simulink model "Practica2OscarModel"  (R2018a)
settings: Solver=VariableStepAuto  StartTime=0.0  StopTime=10.0  RelTol=1e-3  EnableMultiTasking=on
values from neighbouring files (symbols this model uses):
  K = 1.1    [Practica2Oscar.m]    (also in proyectoAvilaSilva.m = Kp/limite; proyectoAvilaSilva2.m = Kp/limite)
  Kd = Kv/lim    [P5OscarAvilaControlDigital.m]    (also in Practica2Oscar.m = 0.22; practica5.m = Kv/double(limit(f,s,0)))
  Kdv = 0.2    [Practica2Oscar.m]
  Ki = K*T/Ti    (= 0.2)    [Practica2Oscar.m]
  Kiv = 1.1    [Practica2Oscar.m]
  Kp = K-Ki/2    (= 1)    [Practica2Oscar.m]    (also in proyectoAvilaSilva.m = 9; proyectoAvilaSilva2.m = 9)
  Kpv = 5.5    [Practica2Oscar.m]
  T = 2.5    [P4OscarAvilaControlDigital.m]    (also in Practica2Oscar.m = 1; practica5.m = 0.02; proyectoAvilaSilva.m = 0.01; proyectoAvilaSilva2.m = 0.01)
  Td = 0.2    [Practica2Oscar.m]
  Ti = 5.5    [Practica2Oscar.m]
libraries: simulink x1
settings Model: Creator=CltControl  LastModifiedBy=sasm
settings OptimizationCC: LifeSpan=inf
settings DebuggingCC: SFUnexpectedBacktrackingDiag=warning  SFNoUnconditionalDefaultTransitionDiag=warning  SFExecutionAtInitializationDiag=none
settings CodeAppCC: StateflowObjectComments=on
settings GRTTargetCC: TargetLangStandard=C89/C90 (ANSI)  GeneratePreprocessorConditionals=Disable all
settings ConfigComp: CovMetricSettings=dw  CovHtmlReporting=on  CovSaveCumulativeToWorkspaceVar=on  CovSaveSingleToWorkspaceVar=on  CovExternalEMLEnable=off

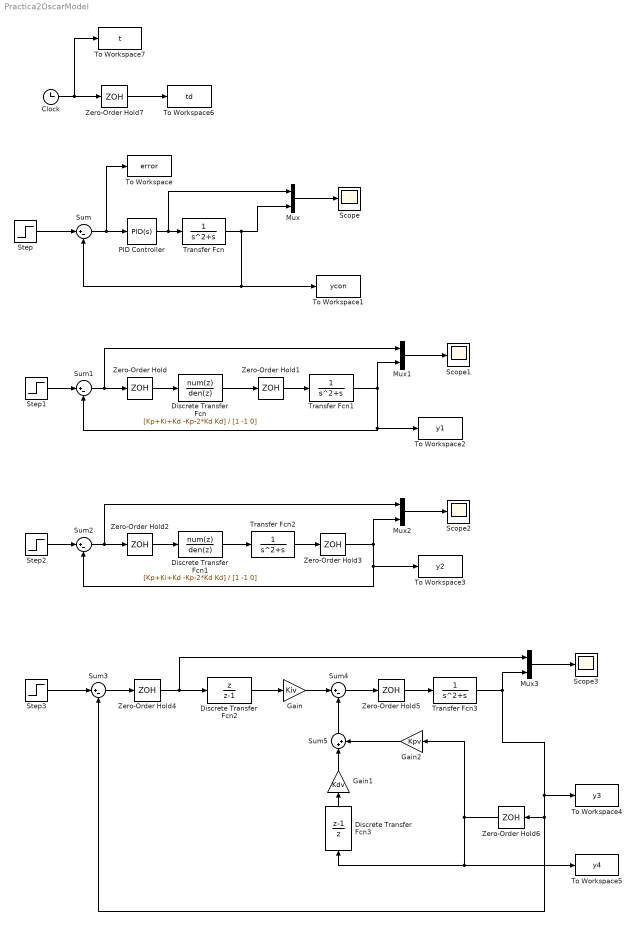
== system Practica2OscarModel ==
  Clock : Clock
  Discrete Transfer Fcn : DiscreteTransferFcn  Numerator=[Kp+Ki+Kd -Kp-2*Kd Kd]  Denominator=[1 -1 0]
  Discrete Transfer Fcn1 : DiscreteTransferFcn  Numerator=[Kp+Ki+Kd -Kp-2*Kd Kd]  Denominator=[1 -1 0]
  Discrete Transfer Fcn2 : DiscreteTransferFcn  Numerator=[1 0]  Denominator=[1 -1]
  Discrete Transfer Fcn3 : DiscreteTransferFcn  Numerator=[1 -1]  Denominator=[1 0]
  Gain : Gain  Gain=Kiv
  Gain1 : Gain  Gain=Kdv
  Gain2 : Gain  Gain=Kpv
  Mux{,1..3} (4 alike) : Mux  Inputs=2
  PID Controller : simulink/Continuous/PID Controller  Controller=PID  TimeDomain=Continuous-time  SampleTime=-1  IntegratorMethod=Forward Euler  FilterMethod=Forward Euler  Form=Ideal  UseFilter=on  ControllerParametersSource=internal  P=K  I=1/Ti  D=Td  N=100  InitialConditionSource=internal  InitialConditionForIntegrator=0  InitialConditionForFilter=0  ExternalReset=none  LimitOutput=off  UpperSaturationLimit=inf  LowerSaturationLimit=-inf  LinearizeAsGain=on  AntiWindupMode=none  Kb=1  TrackingMode=off  Kt=1  PParamMin=[]  PParamMax=[]  IParamMin=[]  IParamMax=[]  DParamMin=[]  DParamMax=[]  NParamMin=[]  NParamMax=[]  KbParamMin=[]  KbParamMax=[]  KtParamMin=[]  KtParamMax=[]  POutMin=[]  POutMax=[]  IOutMin=[]  IOutMax=[]  DOutMin=[]  DOutMax=[]  NOutMin=[]  NOutMax=[]  KbOutMin=[]  KbOutMax=[]  KtOutMin=[]  KtOutMax=[]  IntegratorOutMin=[]  IntegratorOutMax=[]  FilterOutMin=[]  FilterOutMax=[]  SumOutMin=[]  SumOutMax=[]  SumI1OutMin=[]  SumI1OutMax=[]  SumI2OutMin=[]  SumI2OutMax=[]  SumI3OutMin=[]  SumI3OutMax=[]  SumDOutMin=[]  SumDOutMax=[]  SaturationOutMin=[]  SaturationOutMax=[]  IntegratorContinuousStateAttributes=''  IntegratorStateMustResolveToSignalObject=off  IntegratorRTWStateStorageClass=Auto  FilterContinuousStateAttributes=''  FilterStateMustResolveToSignalObject=off  FilterRTWStateStorageClass=Auto  DifferentiatorICPrevScaledInput=0  DifferentiatorOutMin=[]  DifferentiatorOutMax=[]  FilterDiffOutCoefMin=[]  FilterDiffOutCoefMax=[]  SumDenOutMin=[]  SumDenOutMax=[]  SumNumOutMin=[]  SumNumOutMax=[]  ReciprocalOutMin=[]  ReciprocalOutMax=[]  DivideOutMin=[]  DivideOutMax=[]  TunerSelectOption=Transfer Function Based (PID Tuner App)
  Scope{,1..3} (4 alike) : Scope
  Step{,1..3} (4 alike) : Step  SampleTime=0
  Sum{,1..4} (5 alike) : Sum  Inputs=|+-
  Sum5 : Sum  Inputs=|++
  To Workspace : ToWorkspace  VariableName=error  SampleTime=-1
  To Workspace1 : ToWorkspace  VariableName=ycon  SampleTime=-1
  To Workspace2 : ToWorkspace  VariableName=y1  SampleTime=-1
  To Workspace3 : ToWorkspace  VariableName=y2  SampleTime=-1
  To Workspace4 : ToWorkspace  VariableName=y3  SampleTime=-1
  To Workspace5 : ToWorkspace  VariableName=y4  SampleTime=-1
  To Workspace6 : ToWorkspace  VariableName=td  SampleTime=-1
  To Workspace7 : ToWorkspace  VariableName=t  SampleTime=-1
  Transfer Fcn{,1..3} (4 alike) : TransferFcn  Denominator=[1 1 0]
  Zero-Order Hold{,1..7} (8 alike) : ZeroOrderHold  SampleTime=T
  wires:
  Step/1 -> Sum/1
  Sum/1 -> To Workspace/1, PID Controller/1
  PID Controller/1 -> Mux/1, Transfer Fcn/1
  Transfer Fcn/1 -> Sum/2, To Workspace1/1, Mux/2
  Mux/1 -> Scope/1
  Step1/1 -> Sum1/1
  Sum1/1 -> Mux1/1, Zero-Order Hold/1
  Zero-Order Hold/1 -> Discrete Transfer Fcn/1
  Discrete Transfer Fcn/1 -> Zero-Order Hold1/1
  Zero-Order Hold1/1 -> Transfer Fcn1/1
  Mux1/1 -> Scope1/1
  Transfer Fcn1/1 -> Sum1/2, To Workspace2/1, Mux1/2
  Step2/1 -> Sum2/1
  Sum2/1 -> Mux2/1, Zero-Order Hold2/1
  Zero-Order Hold2/1 -> Discrete Transfer Fcn1/1
  Mux2/1 -> Scope2/1
  Transfer Fcn2/1 -> Zero-Order Hold3/1
  Discrete Transfer Fcn1/1 -> Transfer Fcn2/1
  Zero-Order Hold3/1 -> Mux2/2, Sum2/2, To Workspace3/1
  Step3/1 -> Sum3/1
  Sum3/1 -> Zero-Order Hold4/1
  Zero-Order Hold4/1 -> Mux3/1, Discrete Transfer Fcn2/1
  Discrete Transfer Fcn2/1 -> Gain/1
  Gain/1 -> Sum4/1
  Sum4/1 -> Zero-Order Hold5/1
  Zero-Order Hold5/1 -> Transfer Fcn3/1
  Mux3/1 -> Scope3/1
  Transfer Fcn3/1 -> Sum3/2, Zero-Order Hold6/1, To Workspace4/1, Mux3/2
  Sum5/1 -> Sum4/2
  Gain1/1 -> Sum5/1
  Gain2/1 -> Sum5/2
  Discrete Transfer Fcn3/1 -> Gain1/1
  Zero-Order Hold6/1 -> Gain2/1, To Workspace5/1, Discrete Transfer Fcn3/1
  Clock/1 -> To Workspace7/1, Zero-Order Hold7/1
  Zero-Order Hold7/1 -> To Workspace6/1
